simulink model "OFDMTxRx2211"  (R2017b)
settings: Solver=VariableStepAuto  StartTime=0.0  StopTime=10.0  RelTol=1e-3
InitFcn:
  | Ts = 1e-6;
  | simParams.Ts = Ts;
  | simParams.TsTx = Ts;
  | simParams.TsRx = Ts;
  | simParams.nFFT = 1024;
  | simParams.lengthCP = 128;
  | nFFT = simParams.nFFT;
  | simParams.NSubcarriers = 398;
  | simParams.windowing = 16;
undefined symbols (not defined in the file): fft_size, i
libraries: hdlsllib x49, simulink x39, simulink_need_slupdate x12, dspmathops x4, dspxfrm3 x3, dspsigops x2, commdigbbndam3 x1, commseqgen3 x1
(part 1 of 3)
settings Model: PauseTimes=1  NumberOfSteps=100  Creator=Pigrit  LastModifiedBy=trainee

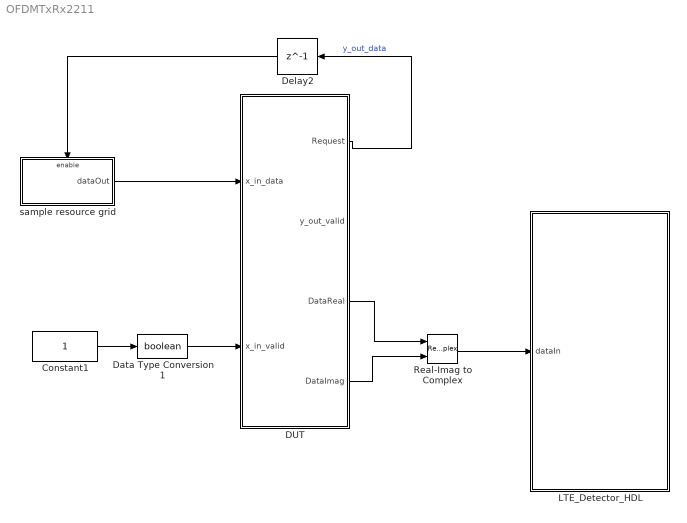
== system OFDMTxRx2211 ==
  Constant1 : Constant  OutDataTypeStr=boolean  SampleTime=simParams.Ts
  DUT : Subsystem  TreatAsAtomicUnit=on
  Data Type Conversion1 : DataTypeConversion  OutDataTypeStr=boolean
  Delay2 : Delay  DelayLength=1  InitialCondition=0  InputProcessing=Columns as channels (frame based)
  LTE_Detector_HDL : Subsystem
  Real-Imag to Complex : RealImagToComplex
  sample resource grid : Subsystem
  wires:
  DUT/3(DataReal) -> Real-Imag to Complex/1
  Delay2/1 -> sample resource grid/Enable
  Data Type Conversion1/1 -> DUT/2(x_in_valid)
  Constant1/1 -> Data Type Conversion1/1
  DUT/1(Request) -> Delay2/1  "y_out_data"
  sample resource grid/1(dataOut) -> DUT/1(x_in_data)
  DUT/4(DataImag) -> Real-Imag to Complex/2
  Real-Imag to Complex/1 -> LTE_Detector_HDL/1(dataIn)

== system OFDMTxRx2211/DUT ==
  x_in_data : Inport
  x_in_valid : Inport  Port=2
  "symmetric " : Subsystem
  Request : Outport
  y_out_valid : Outport  Port=2
  DataReal : Outport  Port=3
  DataImag : Outport  Port=4
  wires:
  x_in_valid/1 -> "symmetric "/Enable, y_out_valid/1
  x_in_data/1 -> "symmetric "/1(x_in)
  "symmetric "/1(y_out) -> Request/1
  "symmetric "/2(Data1) -> DataReal/1
  "symmetric "/3(Data2) -> DataImag/1

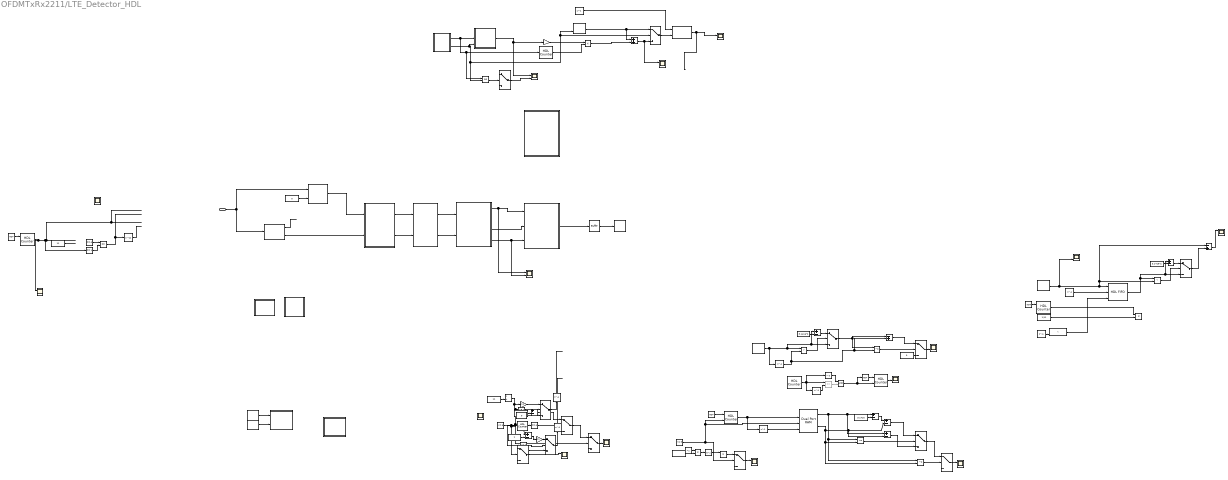
== system OFDMTxRx2211/LTE_Detector_HDL ==
  dataIn : Inport
  Add{,1..4,6,8} (7 alike) : Sum  Inputs=+-
  Add5 : Sum  Inputs=-+
  Add7 : Sum  Inputs=-+
  Add9 : Sum
  AmpAndAngle : Subsystem
  Buffer : Buffer  N=1000  OutputFrames=off
  Compare To Constant : simulink/Logic and Bit Operations/Compare To Constant  relop=>=  const=5  OutDataTypeStr=boolean
  Compare To Constant1 : simulink/Logic and Bit Operations/Compare To Constant  relop===  const=0  OutDataTypeStr=boolean
  Compare To Constant2 : simulink/Logic and Bit Operations/Compare To Constant  relop===  const=1  OutDataTypeStr=boolean
  Compare To Constant3 : simulink/Logic and Bit Operations/Compare To Constant  relop=>=  const=5  OutDataTypeStr=boolean
  Compare To Constant4 : simulink/Logic and Bit Operations/Compare To Constant  relop=>  const=0  OutDataTypeStr=boolean
  Compare To Constant5 : simulink/Logic and Bit Operations/Compare To Constant  relop===  const=0  OutDataTypeStr=boolean
  Compare To Constant6 : simulink/Logic and Bit Operations/Compare To Constant  relop=>=  const=1  OutDataTypeStr=boolean
  Compare To Constant7 : simulink/Logic and Bit Operations/Compare To Constant  relop=>=  const=1  OutDataTypeStr=boolean
  Constant1 : Constant  Value=3.1416  OutDataTypeStr=double  SampleTime=simParams.Ts
  Constant10 : Constant  Value=0  OutDataTypeStr=uint8  SampleTime=simParams.Ts
  Constant11 : Constant  OutDataTypeStr=double  SampleTime=simParams.Ts
  Constant12 : Constant  Value=11  OutDataTypeStr=uint8  SampleTime=simParams.Ts
  Constant2 : Constant  Value=complex(0+i)  SampleTime=simParams.Ts
  Constant3 : Constant  Value=3.1416  OutDataTypeStr=double  SampleTime=simParams.Ts
  Constant4 : Constant  Value=3.1416*2  OutDataTypeStr=double  SampleTime=simParams.Ts
  Constant5 : Constant  Value=0  OutDataTypeStr=double  SampleTime=simParams.Ts
  Constant6 : Constant  Value=1/11  SampleTime=simParams.Ts
  Constant7 : Constant  Value=3.1416*2  OutDataTypeStr=double  SampleTime=simParams.Ts
  Constant8 : Constant  Value=11  OutDataTypeStr=int16  SampleTime=simParams.Ts
  Constant9 : Constant  Value=0  OutDataTypeStr=int8  SampleTime=simParams.Ts
  Constellation Diagram : ConstellationDiagram
  Delay1 : Delay  DelayLength=1  InitialCondition=0  InputProcessing=Columns as channels (frame based)
  Delay{2..3,6..9} (6 alike) : Delay  DelayLength=1  InitialCondition=0  UseCircularBuffer=on
  Delay4 : Delay  DelayLength=1  InitialCondition=0  InputProcessing=Columns as channels (frame based)
  Delay5 : Delay  DelayLength=11  InitialCondition=0  InputProcessing=Columns as channels (frame based)
  Divide : Product  Inputs=*/  OutDataTypeStr=uint8  SaturateOnIntegerOverflow=on  RndMeth=Zero
  Dual Port RAM : hdlsllib/HDL RAMs/Dual Port RAM  ram_size=8
      settings: SourceProductName=HDL Coder  SourceProductBaseCode=HD
  FFT : Subsystem
  Frequency_Correction : Subsystem
  Frequency_Correction1 : Subsystem
  Frequency_Estimation : Subsystem
  Frequency_Estimation1 : Subsystem
  Gain : Gain  Gain=11  OutDataTypeStr=uint8
  Gain1 : Gain  Gain=11  OutDataTypeStr=uint8
  Gain2 : Gain  Gain=1/10
  HDL Counter : hdlsllib/Sources/HDL Counter  CountType=Count limited  CountInit=0  CountStep=1  CountMax=1  CountFromType=Initial value  CountFrom=0  CountResetPort=off  CountLoadPort=off  CountEnbPort=on  CountDirPort=off  CountDataType=Unsigned  CountWordLen=1  CountFracLen=0  CountSampTime=1
      settings: SourceProductBaseCode=HD
  HDL Counter1 : hdlsllib/Sources/HDL Counter  CountType=Count limited  CountInit=1  CountStep=1  CountMax=60  CountFromType=Initial value  CountFrom=1  CountResetPort=on  CountLoadPort=off  CountEnbPort=on  CountDirPort=off  CountDataType=Unsigned  CountWordLen=8  CountFracLen=0  CountSampTime=1
      settings: SourceProductBaseCode=HD
  HDL Counter2 : hdlsllib/Sources/HDL Counter  CountType=Count limited  CountInit=0  CountStep=1  CountMax=60  CountFromType=Initial value  CountFrom=0  CountResetPort=on  CountLoadPort=off  CountEnbPort=on  CountDirPort=off  CountDataType=Unsigned  CountWordLen=8  CountFracLen=0  CountSampTime=1
      settings: SourceProductBaseCode=HD
  HDL Counter3 : hdlsllib/Sources/HDL Counter  CountType=Count limited  CountInit=0  CountStep=1  CountMax=1024  CountFromType=Initial value  CountFrom=0  CountResetPort=on  CountLoadPort=off  CountEnbPort=on  CountDirPort=off  CountDataType=Unsigned  CountWordLen=16  CountFracLen=0  CountSampTime=1
      settings: SourceProductBaseCode=HD
  HDL Counter4 : hdlsllib/Sources/HDL Counter  CountType=Count limited  CountInit=0  CountStep=1  CountMax=40  CountFromType=Initial value  CountFrom=0  CountResetPort=off  CountLoadPort=off  CountEnbPort=on  CountDirPort=off  CountDataType=Unsigned  CountWordLen=8  CountFracLen=0  CountSampTime=1
      settings: SourceProductBaseCode=HD
  HDL Counter5 : hdlsllib/Sources/HDL Counter  CountType=Count limited  CountInit=0  CountStep=1  CountMax=40  CountFromType=Initial value  CountFrom=0  CountResetPort=on  CountLoadPort=off  CountEnbPort=on  CountDirPort=off  CountDataType=Unsigned  CountWordLen=8  CountFracLen=0  CountSampTime=1
      settings: SourceProductBaseCode=HD
  HDL Counter7 : hdlsllib/Sources/HDL Counter  CountType=Count limited  CountInit=0  CountStep=1  CountMax=9  CountFromType=Initial value  CountFrom=0  CountResetPort=off  CountLoadPort=off  CountEnbPort=on  CountDirPort=off  CountDataType=Unsigned  CountWordLen=8  CountFracLen=0  CountSampTime=1
      settings: SourceProductBaseCode=HD
  HDL FIFO : hdlsllib/HDL RAMs/HDL FIFO  fifo_size=40  ratio=1  push_msg=Warning  pop_msg=Warning  show_empty=off  show_full=off  show_num=off
      settings: SourceProductName=HDL Coder  SourceProductBaseCode=HD
  Logical Operator1 : Logic  Operator=NOT  IconShape=distinctive  AllPortsSameDT=off  OutDataTypeStr=boolean
  Logical Operator2 : Logic  Operator=NOT  IconShape=distinctive  AllPortsSameDT=off  OutDataTypeStr=boolean
  Logical Operator3 : Logic  Operator=OR  AllPortsSameDT=off  OutDataTypeStr=boolean
  Logical Operator4 : Logic  Operator=OR  AllPortsSameDT=off  OutDataTypeStr=boolean
  Logical Operator6 : Logic  AllPortsSameDT=off  OutDataTypeStr=boolean
  Logical Operator7 : Logic  Operator=NOT  Inputs=1  AllPortsSameDT=off  OutDataTypeStr=boolean
  Logical Operator8 : Logic  Operator=NOT  AllPortsSameDT=off  OutDataTypeStr=boolean
  Number of subcarriers : Constant  Value=0  OutDataTypeStr=fixdt(0,12,0)  SampleTime=Ts
  Pow : Math  RndMeth=Zero  SaturateOnIntegerOverflow=on
  Product{,1..3} (4 alike) : Product
  Relational Operator : RelationalOperator  Operator=~=  OutDataTypeStr=boolean  RndMeth=Nearest
  Relational Operator1 : RelationalOperator  Operator=<=  OutDataTypeStr=boolean  RndMeth=Nearest
  Relational Operator2 : RelationalOperator  Operator=>  OutDataTypeStr=boolean  RndMeth=Nearest
  Relational Operator3 : RelationalOperator  Operator=~=  OutDataTypeStr=boolean  RndMeth=Nearest
  Relational Operator4 : RelationalOperator  Operator=<  OutDataTypeStr=boolean  RndMeth=Nearest
  Relational Operator5 : RelationalOperator  Commented=on  Operator===  OutDataTypeStr=boolean  RndMeth=Nearest
  Relational Operator6 : RelationalOperator  Operator=<  OutDataTypeStr=boolean  RndMeth=Nearest
  Scope{1..3,5..8,11..15} (12 alike) : Scope  NumInputPorts=2
  Scope10 : Scope  NumInputPorts=3
  Scope4 : Scope
  Scope9 : Scope  NumInputPorts=3
  Subsystem1 : Subsystem
  Subsystem2 : Subsystem
  Switch{1..13} (13 alike) : Switch  Criteria=u2 ~= 0
  Unary Minus : UnaryMinus
  Unit Delay Enabled Synchronous{1..4,6} (5 alike) : hdlsllib/Discrete/Unit Delay Enabled Synchronous  InitialCondition=0.0  SampleTime=-1
      settings: SourceProductName=HDL Coder  SourceProductBaseCode=HD
  Подкрутка фазы1 : Subsystem
  Подстройка фаз по пилотным : Subsystem
  "Рабочая версия с недокрученной фазой " : Subsystem
  Стробирование сигнала на nFFT отсчетов : Subsystem
  Устранение 2pi неопределенности и вычисление разности фаз : Subsystem
  Устранение 2pi неопределенности и вычисление разности фаз2 : Subsystem
  wires:
  Frequency_Estimation1/1(freqEst) -> ?
  Frequency_Correction1/1(dataOut) -> Стробирование сигнала на nFFT отсчетов/1(In1)
  Frequency_Estimation1/2(MiddlePoint) -> Стробирование сигнала на nFFT отсчетов/2(In2)
  Стробирование сигнала на nFFT отсчетов/1(dataOut) -> FFT/1(dataIn)
  Стробирование сигнала на nFFT отсчетов/2(ValidOut) -> FFT/2(validIn)
  Switch1/1 -> Switch2/1
  Switch2/1 -> Scope4/1
  ? -> Switch1/3, Add/1, Switch3/1
  Compare To Constant/1 -> Switch2/2, Switch3/2, HDL Counter/1
  Switch3/1 -> Scope2/1
  Compare To Constant1/1 -> Switch1/2
  Add/1 -> Switch1/1
  Constant1/1 -> Add/2
  HDL Counter/1 -> Compare To Constant1/1
  ? -> Scope2/2, Compare To Constant/1
  Switch7/1 -> Scope1/1
  Pow/1 -> Product1/1
  ? -> Dual Port RAM/1, Unary Minus/1
  ? -> Compare To Constant3/1
  Unary Minus/1 -> Product/1
  Logical Operator2/1 -> HDL Counter2/1
  Add1/1 -> Add2/1
  Relational Operator1/1 -> Switch6/2
  Constant3/1 -> Add1/2
  Add3/1 -> Switch6/3
  Relational Operator/1 -> Switch7/2
  Compare To Constant3/1 -> Dual Port RAM/3, HDL Counter2/2, Switch5/2
  Add2/1 -> Switch6/1
  Delay2/1 -> Dual Port RAM/4
  Constant2/1 -> Product/2
  Switch5/1 -> Scope3/1
  ? -> Product1/2
  Dual Port RAM/2 -> Relational Operator1/2, Relational Operator/2, Add3/2, Add2/2
  Dual Port RAM/1 -> Add3/1, Add1/1, Relational Operator1/1, Relational Operator/1
  Product1/1 -> Switch5/1
  Switch6/1 -> Switch7/1
  HDL Counter2/1 -> Dual Port RAM/2, Delay2/1
  ? -> Logical Operator2/1, Scope3/2
  Product/1 -> Pow/1
  FFT/1(dataOut) -> AmpAndAngle/1(In1)
  FFT/2(validOut) -> AmpAndAngle/2(In2)
  Logical Operator6/1 -> Logical Operator7/1, HDL Counter5/2
  Relational Operator5/1 -> Logical Operator6/2
  Compare To Constant4/1 -> Logical Operator6/1
  Delay6/1 -> Relational Operator5/2
  HDL Counter4/1 -> Compare To Constant4/1, Relational Operator5/1, Delay6/1
  Switch9/1 -> Scope5/2
  Switch8/1 -> Add5/1, Relational Operator3/1
  Constant5/1 -> Switch9/3
  Unit Delay Enabled Synchronous1/1 -> Add4/1, Switch8/3, Relational Operator2/1, Delay3/1
  Relational Operator3/1 -> Switch9/2
  Relational Operator2/1 -> Switch8/2
  Constant4/1 -> Add4/2
  Logical Operator7/1 -> HDL Counter5/1
  Add4/1 -> Switch8/1
  Add5/1 -> Switch9/1
  HDL Counter5/1 -> Scope7/2
  ? -> HDL Counter4/1, Unit Delay Enabled Synchronous1/2
  Delay3/1 -> Add5/2, Relational Operator3/2, Relational Operator2/2
  ? -> Delay1/1
  HDL FIFO/1 -> Add6/1, Switch4/3, Relational Operator6/1
  ? -> Unit Delay Enabled Synchronous2/2
  Logical Operator1/1 -> HDL Counter1/1
  ? -> Unit Delay Enabled Synchronous2/1
  Constant7/1 -> Add6/2
  Relational Operator6/1 -> Switch4/2
  Add7/1 -> Scope6/1
  ? -> Scope6/2
  ? -> HDL Counter1/2
  Add6/1 -> Switch4/1
  Delay1/1 -> Relational Operator4/2
  Constant6/1 -> Product2/2
  Unit Delay Enabled Synchronous2/1 -> Scope8/2, Add7/1, Relational Operator6/2, HDL FIFO/1
  ? -> Relational Operator4/1
  ? -> Delay4/1
  Switch4/1 -> Add7/2
  Delay4/1 -> HDL FIFO/2
  HDL Counter1/1 -> Product2/1
  Relational Operator4/1 -> HDL FIFO/3
  Unit Delay Enabled Synchronous3/1 -> Устранение 2pi неопределенности и вычисление разности фаз/2("Фаза \"правого\" пилота")
  Unit Delay Enabled Synchronous4/1 -> Устранение 2pi неопределенности и вычисление разности фаз/1("Фаза \"левого\" пилота")
  ? -> Unit Delay Enabled Synchronous3/1
  ? -> Unit Delay Enabled Synchronous4/1
  Constant8/1 -> ?
  ? -> Compare To Constant5/1
  Compare To Constant2/1 -> Logical Operator3/2
  ? -> Logical Operator8/1, Scope10/2, HDL Counter3/2
  ? -> ?
  Delay5/1 -> ?
  ? -> Scope9/1
  Logical Operator8/1 -> HDL Counter3/1
  Logical Operator3/1 -> Delay5/1
  HDL Counter3/1 -> Scope10/1, Compare To Constant2/1
  Compare To Constant5/1 -> Logical Operator3/1
  Delay7/1 -> ?
  Add8/1 -> Gain1/1
  Compare To Constant6/1 -> Switch10/2
  Gain/1 -> Switch10/1
  Constant9/1 -> Switch10/3
  Switch11/1 -> Delay7/1
  Delay8/1 -> ?
  Constant10/1 -> Switch11/3
  Constant12/1 -> Divide/2
  ? -> Divide/1
  Divide/1 -> Gain/1, Add8/1, Compare To Constant7/1, Compare To Constant6/1
  Constant11/1 -> Add8/2
  Compare To Constant7/1 -> Switch11/2
  Switch10/1 -> Delay8/1
  Gain1/1 -> Switch11/1
  ? -> Delay9/1
  Подкрутка фазы1/1(Out1) -> Scope12/1
  Add9/1 -> Scope15/1, Switch12/3
  Gain2/1 -> Product3/1
  Unit Delay Enabled Synchronous6/1 -> Add9/1, Switch12/1
  Subsystem2/1("Passe diff ") -> Scope13/1, Gain2/1
  Subsystem1/2(IndexPilot) -> Logical Operator4/2, Unit Delay Enabled Synchronous6/2, Switch12/2, Subsystem2/3("Index Pil ")
  Subsystem1/1(InformIndex) -> Logical Operator4/1, HDL Counter7/1, Subsystem2/2(Index Inf)
  Delay9/1 -> Подкрутка фазы1/1(PuuuSii)
  HDL Counter7/1 -> Product3/2
  ? -> Switch13/1, Unit Delay Enabled Synchronous6/1, Subsystem2/1(Pilot Phase)
  Switch13/1 -> Scope13/2
  Product3/1 -> Add9/2
  Logical Operator4/1 -> Switch13/2
  Switch12/1 -> Подкрутка фазы1/2("DifPhase ")
  Buffer/1 -> Constellation Diagram/1
  AmpAndAngle/3(AngOut) -> Подстройка фаз по пилотным/2(AngIn)
  AmpAndAngle/4(ValidOut) -> Scope14/2, Подстройка фаз по пилотным/3("ValidIn ")
  Подстройка фаз по пилотным/1(Out1) -> Buffer/1
  AmpAndAngle/1("PureSig ") -> Scope14/1, Подстройка фаз по пилотным/1(PureSigIn)
  dataIn/1 -> Frequency_Correction1/1(dataIn), Frequency_Estimation1/1(data)
  Number of subcarriers/1 -> Frequency_Correction1/2(freq)

== system OFDMTxRx2211/sample resource grid ==
  request1 : EnablePort
  PN Sequence Generator : commseqgen3/PN Sequence Generator  poly='z^23+z^21+z^17 + z^11 + z^5 +1'  ini_sta=[0 1 1 0 0 1 0 0 0 0 1 0 1 1 0 0 1 0 0 1 0 0 1]  outBitMaskSource=Dialog parameter  shift=0  outVarSiz=off  maxOutSizeMode=Dialog parameter  maxOutSize=[10 1]  Ts=simParams.Ts  sampPerFrame=1  reset=off  bitPackedOutputs=on  outDataType=boolean  numPackedBits=2  bitPackDataSigned=off  bitPackedOutDType=Smallest integer
      settings: SourceProductName=Communications System Toolbox
  dataOut : Outport
  wires:
  PN Sequence Generator/1 -> dataOut/1

== system OFDMTxRx2211/DUT/symmetric  ==
  x_in : Inport
  Enable : EnablePort
  Add CP and windowing : Subsystem
  Complex to Real-Imag : ComplexToRealImag
  IFFT : Subsystem
  Scope : Scope  NumInputPorts=2
  Scope1 : Scope  NumInputPorts=2
  fORM1 : Subsystem
  y_out1 : Scope  NumInputPorts=2
  "Сдвиг в симметричный вид " : Subsystem
  y_out : Outport  InitialOutput=0
  Data1 : Outport  Port=2  InitialOutput=0
  Data2 : Outport  Port=3  InitialOutput=0
  wires:
  fORM1/1(dataRequest) -> y_out/1
  x_in/1 -> fORM1/1(dataIn)
  Add CP and windowing/1(Out1) -> Complex to Real-Imag/1
  Complex to Real-Imag/1 -> Data2/1
  IFFT/1(dataOut) -> Scope/1, Add CP and windowing/1(In1)
  Complex to Real-Imag/2 -> Data1/1
  "Сдвиг в симметричный вид "/1(dataOut) -> Scope1/1, IFFT/1(dataIn)
  "Сдвиг в симметричный вид "/2(validOut) -> Scope1/2, IFFT/2(validIn)
  IFFT/2(validOut) -> Scope/2, Add CP and windowing/2(In2)
  fORM1/2(dataOut) -> y_out1/1, "Сдвиг в симметричный вид "/1(dataIn)
  fORM1/3(validOut) -> y_out1/2, "Сдвиг в симметричный вид "/2(validIn)

== system OFDMTxRx2211/LTE_Detector_HDL/AmpAndAngle ==
  In1 : Inport
  In2 : Inport  Port=2
  Compare To Constant2 : simulink/Logic and Bit Operations/Compare To Constant  relop=<  const=512  OutDataTypeStr=boolean
  Delay1 : Delay  DelayLength=512  InitialCondition=0  InputProcessing=Columns as channels (frame based)
  Delay2 : Delay  DelayLength=22  InitialCondition=0  InputProcessing=Columns as channels (frame based)
  Delay4 : Delay  DelayLength=1024  InitialCondition=0  InputProcessing=Columns as channels (frame based)
  HDL Counter1 : hdlsllib/Sources/HDL Counter  CountType=Count limited  CountInit=0  CountStep=1  CountMax=1023  CountFromType=Initial value  CountFrom=0  CountResetPort=on  CountLoadPort=off  CountEnbPort=on  CountDirPort=off  CountDataType=Unsigned  CountWordLen=11  CountFracLen=0  CountSampTime=1
      settings: SourceProductBaseCode=HD
  Logical Operator1 : Logic  Operator=NOT  IconShape=distinctive  AllPortsSameDT=off  OutDataTypeStr=boolean
  Rect_to_Polar : Subsystem
  Signal Specification1 : SignalSpecification  Dimensions=1
  Switch4 : Switch  Criteria=u2 ~= 0
  "PureSig " : Outport
  MagOut : Outport  Port=2
  AngOut : Outport  Port=3
  ValidOut : Outport  Port=4
  wires:
  Delay4/1 -> Switch4/3
  Compare To Constant2/1 -> Switch4/2
  HDL Counter1/1 -> Compare To Constant2/1
  Logical Operator1/1 -> HDL Counter1/1
  Switch4/1 -> Delay2/1, Signal Specification1/1
  Delay1/1 -> Logical Operator1/1, HDL Counter1/2, Rect_to_Polar/2("ValidIn ")
  In2/1 -> Delay1/1
  In1/1 -> Switch4/1, Delay4/1
  Rect_to_Polar/3(validOut) -> ValidOut/1
  Rect_to_Polar/1(magOut) -> MagOut/1
  Delay2/1 -> "PureSig "/1
  Rect_to_Polar/2(angleOut) -> AngOut/1
  Signal Specification1/1 -> Rect_to_Polar/1(dataIn)

== system OFDMTxRx2211/LTE_Detector_HDL/FFT ==
  note: Set input of FFT to input wordlength + FFT growth to allow
      | the output of the FFT to scale. Maximum bit growth is equal
      | to log2(nFFT).
  dataIn : Inport
  validIn : Inport  Port=2
  Data Type Conversion : DataTypeConversion  OutDataTypeStr=fixdt(1,18,10)  RndMeth=Round
  Delay{1..2,4..5} (4 alike) : Delay  DelayLength=1  InitialCondition=0  InputProcessing=Columns as channels (frame based)
  FFT HDL Optimized : dspxfrm3/FFT HDL Optimized  FFTLength=1024  Architecture=Streaming Radix 2^2  ComplexMultiplication=Use 3 multipliers and 5 adders  BitReversedOutput=off  BitReversedInput=off  Normalize=off  SimulateUsing=Code generation  RoundingMethod=Floor  ResetInputPort=off  StartOutputPort=off  EndOutputPort=off
      settings: SourceProductName=DSP System Toolbox  SourceProductBaseCode=DS
  Signal Specification : SignalSpecification  Dimensions=1
  Signal Specification1 : SignalSpecification  Dimensions=1
  dataOut : Outport
  validOut : Outport  Port=2
  wires:
  Signal Specification1/1 -> FFT HDL Optimized/2
  Signal Specification/1 -> FFT HDL Optimized/1
  FFT HDL Optimized/2 -> Delay5/1
  FFT HDL Optimized/1 -> Delay4/1
  Delay4/1 -> Data Type Conversion/1
  Delay2/1 -> Signal Specification1/1
  dataIn/1 -> Delay1/1
  validIn/1 -> Delay2/1
  Delay1/1 -> Signal Specification/1
  Data Type Conversion/1 -> dataOut/1
  Delay5/1 -> validOut/1

== system OFDMTxRx2211/LTE_Detector_HDL/Frequency_Correction ==
  note: This subsystem corrects the frequency offset using an Numerically Controller Oscillator (NCO) and a conjugate multiplication.
  dataIn : Inport
  freq : Inport  Port=2
  Data Type Conversion : DataTypeConversion  OutDataTypeStr=fixdt(1,16,15)  RndMeth=Nearest
  Delay{1..6} (6 alike) : Delay  DelayLength=1  InitialCondition=0  UseCircularBuffer=on
  Gain : Gain  Gain=2^9  OutDataTypeStr=int16
  NCO HDL Optimized : dspsigops/NCO HDL Optimized  PhaseIncrementSource=Input port  PhaseIncrement=100  PhaseOffsetSource=Property  PhaseOffset=0  DitherSource=Property  NumDitherBits=4  PhaseQuantization=on  NumQuantizerAccumulatorBits=12  LUTCompress=on  ResetAction=off  ValidInputPort=off  Waveform=Complex exponential  PhasePort=off  SimulateUsing=Code generation  AccumulatorWL=16  OutputDataType=Binary point scaling  OutputWL=16  OutputFL=14
      settings: SourceProductName=DSP System Toolbox  SourceProductBaseCode=DS
  Product1 : Product
  Scope : Scope  NumInputPorts=2
  Signal Spec : SignalSpecification  Dimensions=1
  Unit Delay Enabled : simulink_need_slupdate/Unit Delay Enabled  vinit=0.0  tsamp=-1
      settings: SourceProductName=Simulink  SourceProductBaseCode=SL
  complexConjugate : Math  Operator=conj  SaturateOnIntegerOverflow=on
  dataOut : Outport
  wires:
  complexConjugate/1 -> Delay3/1
  NCO HDL Optimized/2 -> Unit Delay Enabled/2
  dataIn/1 -> Delay2/1
  Product1/1 -> Delay4/1
  NCO HDL Optimized/1 -> Unit Delay Enabled/1
  Unit Delay Enabled/1 -> complexConjugate/1
  Data Type Conversion/1 -> Delay1/1
  Delay2/1 -> Scope/2, Product1/1
  Delay1/1 -> dataOut/1
  Delay4/1 -> Data Type Conversion/1
  Delay3/1 -> Scope/1, Product1/2
  Gain/1 -> Delay5/1
  freq/1 -> Delay6/1
  Delay6/1 -> Gain/1
  Signal Spec/1 -> NCO HDL Optimized/1
  Delay5/1 -> Signal Spec/1

== system OFDMTxRx2211/LTE_Detector_HDL/Frequency_Correction1 ==
  note: This subsystem corrects the frequency offset using an Numerically Controller Oscillator (NCO) and a conjugate multiplication.
  dataIn : Inport
  freq : Inport  Port=2
  Data Type Conversion : DataTypeConversion  OutDataTypeStr=fixdt(1,16,15)  RndMeth=Nearest
  Delay{1..6} (6 alike) : Delay  DelayLength=1  InitialCondition=0  UseCircularBuffer=on
  Gain : Gain  Gain=2^9  OutDataTypeStr=int16
  NCO HDL Optimized : dspsigops/NCO HDL Optimized  PhaseIncrementSource=Input port  PhaseIncrement=100  PhaseOffsetSource=Property  PhaseOffset=0  DitherSource=Property  NumDitherBits=4  PhaseQuantization=on  NumQuantizerAccumulatorBits=12  LUTCompress=on  ResetAction=off  ValidInputPort=off  Waveform=Complex exponential  PhasePort=off  SimulateUsing=Code generation  AccumulatorWL=16  OutputDataType=Binary point scaling  OutputWL=16  OutputFL=14
      settings: SourceProductName=DSP System Toolbox  SourceProductBaseCode=DS
  Product1 : Product
  Scope : Scope  NumInputPorts=2
  Signal Spec : SignalSpecification  Dimensions=1
  Unit Delay Enabled : simulink_need_slupdate/Unit Delay Enabled  vinit=0.0  tsamp=-1
      settings: SourceProductName=Simulink  SourceProductBaseCode=SL
  complexConjugate : Math  Operator=conj  SaturateOnIntegerOverflow=on
  dataOut : Outport
  wires:
  complexConjugate/1 -> Delay3/1
  NCO HDL Optimized/2 -> Unit Delay Enabled/2
  dataIn/1 -> Delay2/1
  Product1/1 -> Delay4/1
  NCO HDL Optimized/1 -> Unit Delay Enabled/1
  Unit Delay Enabled/1 -> complexConjugate/1
  Data Type Conversion/1 -> Delay1/1
  Delay2/1 -> Scope/2, Product1/1
  Delay1/1 -> dataOut/1
  Delay4/1 -> Data Type Conversion/1
  Delay3/1 -> Scope/1, Product1/2
  Gain/1 -> Delay5/1
  freq/1 -> Delay6/1
  Delay6/1 -> Gain/1
  Signal Spec/1 -> NCO HDL Optimized/1
  Delay5/1 -> Signal Spec/1

== system OFDMTxRx2211/LTE_Detector_HDL/Frequency_Estimation ==
  data : Inport
  Angle_Filter : Subsystem
  Angle_at_Maximum : Subsystem
  Cyclic_Prefix_Correlator : Subsystem
  Delay14 : Delay  DelayLength=30  InitialCondition=0  UseCircularBuffer=on
  Rect_to_Polar : Subsystem
  Scope1 : Scope  NumInputPorts=2
  freqEst : Outport
  MiddlePoint : Outport  Port=2
  wires:
  Angle_at_Maximum/1(angleOut) -> Angle_Filter/1(angleIn)
  Cyclic_Prefix_Correlator/1(corrOut) -> Scope1/2, Rect_to_Polar/1(dataIn)
  Angle_at_Maximum/2(validOut) -> Delay14/1, MiddlePoint/1, Angle_Filter/2(en)
  Angle_Filter/1(angleOut) -> freqEst/1
  data/1 -> Cyclic_Prefix_Correlator/1(dataIn)
  Delay14/1 -> Scope1/1
  Rect_to_Polar/1(magOut) -> Angle_at_Maximum/1(MagIn)
  Rect_to_Polar/2(angleOut) -> Angle_at_Maximum/2(AngleIn)
  Rect_to_Polar/3(validOut) -> Angle_at_Maximum/3(ValidIn)

== system OFDMTxRx2211/LTE_Detector_HDL/Frequency_Estimation1 ==
  data : Inport
  Angle_Filter : Subsystem
  Angle_at_Maximum : Subsystem
  Cyclic_Prefix_Correlator : Subsystem
  Delay14 : Delay  DelayLength=30  InitialCondition=0  UseCircularBuffer=on
  Rect_to_Polar : Subsystem
  Scope1 : Scope  NumInputPorts=2
  freqEst : Outport
  MiddlePoint : Outport  Port=2
  wires:
  Rect_to_Polar/3(validOut) -> Angle_at_Maximum/3(validIn)
  Angle_at_Maximum/1(angleOut) -> Angle_Filter/1(angleIn)
  Rect_to_Polar/1(magOut) -> Angle_at_Maximum/1(magIn)
  Cyclic_Prefix_Correlator/1(corrOut) -> Scope1/2, Rect_to_Polar/1(dataIn)
  Angle_at_Maximum/2(ValidOut) -> Delay14/1, MiddlePoint/1, Angle_Filter/2(en)
  Rect_to_Polar/2(angleOut) -> Angle_at_Maximum/2(angleIn)
  Angle_Filter/1(angleOut) -> freqEst/1
  data/1 -> Cyclic_Prefix_Correlator/1(dataIn)
  Delay14/1 -> Scope1/1

== system OFDMTxRx2211/LTE_Detector_HDL/Subsystem1 ==
  In1 : Inport
  AND : Logic  IconShape=distinctive  AllPortsSameDT=off  OutDataTypeStr=boolean
  Abs : Abs
  Add6 : Sum  Inputs=+-  OutDataTypeStr=fixdt(1,16,0)
  Compare To Constant5 : simulink/Logic and Bit Operations/Compare To Constant  relop===  const=1  OutDataTypeStr=boolean
  Compare To Zero : simulink/Logic and Bit Operations/Compare To Zero  relop=~=  OutDataTypeStr=boolean
  Constant6 : Constant  Value=11  OutDataTypeStr=int16  SampleTime=simParams.Ts
  FFT Size : Constant  Value=nFFT  OutDataTypeStr=fixdt(0,ceil(log2(simParams.nFFT))+1,0)  SampleTime=Ts
  FFT Size / 2 : ArithShift  BitShiftNumber=1  BitShiftDirection=Right
  HDL Counter3 : hdlsllib/Sources/HDL Counter  CountType=Count limited  CountInit=0  CountStep=1  CountMax=1023  CountFromType=Initial value  CountFrom=0  CountResetPort=off  CountLoadPort=off  CountEnbPort=on  CountDirPort=off  CountDataType=Unsigned  CountWordLen=11  CountFracLen=0  CountSampTime=1
      settings: SourceProductBaseCode=HD
  Logical Operator : Logic  AllPortsSameDT=off  OutDataTypeStr=boolean
  Logical Operator3 : Logic  Operator=NOT  Inputs=1  AllPortsSameDT=off  OutDataTypeStr=boolean
  Logical Operator4 : Logic  AllPortsSameDT=off  OutDataTypeStr=boolean
  Math Function : Math  Operator=mod  RndMeth=Zero  SaturateOnIntegerOverflow=on
  NSubcarriers / 2 : ArithShift  BitShiftNumber=1  BitShiftDirection=Right
  Number of subcarriers : Constant  Value=simParams.NSubcarriers  OutDataTypeStr=fixdt(0,12,0)  SampleTime=Ts
  Relational Operator4 : RelationalOperator  Operator=<=  OutDataTypeStr=boolean  RndMeth=Nearest
  InformIndex : Outport
  IndexPilot : Outport  Port=2
  wires:
  In1/1 -> HDL Counter3/1
  HDL Counter3/1 -> Add6/2
  FFT Size/1 -> FFT Size / 2/1
  Logical Operator/1 -> InformIndex/1
  Constant6/1 -> Math Function/2
  AND/1 -> Logical Operator4/2, Logical Operator/2
  Number of subcarriers/1 -> NSubcarriers / 2/1
  Add6/1 -> Abs/1
  Logical Operator3/1 -> Logical Operator/1
  Abs/1 -> Relational Operator4/1, Compare To Zero/1, Math Function/1
  NSubcarriers / 2/1 -> Relational Operator4/2
  FFT Size / 2/1 -> Add6/1
  Compare To Zero/1 -> AND/1
  Math Function/1 -> Compare To Constant5/1
  Relational Operator4/1 -> AND/2
  Logical Operator4/1 -> IndexPilot/1
  Compare To Constant5/1 -> Logical Operator4/1, Logical Operator3/1

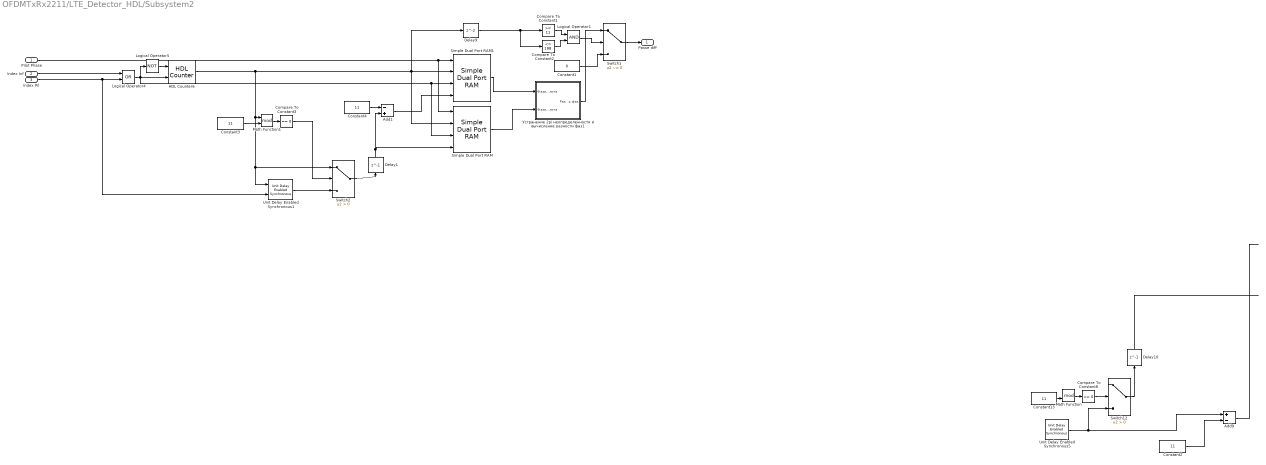
== system OFDMTxRx2211/LTE_Detector_HDL/Subsystem2 ==
  Pilot Phase : Inport
  Index Inf : Inport  Port=2
  "Index Pil " : Inport  Port=3
  Add1 : Sum  Inputs=-+
  Add9 : Sum  Inputs=+-
  Compare To Constant1 : simulink/Logic and Bit Operations/Compare To Constant  relop=>=  const=11  OutDataTypeStr=boolean
  Compare To Constant2 : simulink/Logic and Bit Operations/Compare To Constant  relop=<=  const=198  OutDataTypeStr=boolean
  Compare To Constant3 : simulink/Logic and Bit Operations/Compare To Constant  relop===  const=0  OutDataTypeStr=boolean
  Compare To Constant8 : simulink/Logic and Bit Operations/Compare To Constant  relop===  const=0  OutDataTypeStr=boolean
  Constant1 : Constant  Value=0  OutDataTypeStr=uint8  SampleTime=simParams.Ts
  Constant{2..4,13} (4 alike) : Constant  Value=11  OutDataTypeStr=uint8  SampleTime=simParams.Ts
  Delay1 : Delay  DelayLength=1  InitialCondition=0  UseCircularBuffer=on
  Delay10 : Delay  DelayLength=1  InitialCondition=0  UseCircularBuffer=on
  Delay9 : Delay  InitialCondition=0  UseCircularBuffer=on
  HDL Counter6 : hdlsllib/Sources/HDL Counter  CountType=Count limited  CountInit=0  CountStep=1  CountMax=255  CountFromType=Initial value  CountFrom=0  CountResetPort=on  CountLoadPort=off  CountEnbPort=on  CountDirPort=off  CountDataType=Unsigned  CountWordLen=8  CountFracLen=0  CountSampTime=1
      settings: SourceProductBaseCode=HD
  Logical Operator1 : Logic  AllPortsSameDT=off  OutDataTypeStr=boolean
  Logical Operator4 : Logic  Operator=OR  AllPortsSameDT=off  OutDataTypeStr=boolean
  Logical Operator5 : Logic  Operator=NOT  AllPortsSameDT=off  OutDataTypeStr=boolean
  Math Function : Math  Operator=mod  RndMeth=Zero  SaturateOnIntegerOverflow=on
  Math Function1 : Math  Operator=mod  RndMeth=Zero  SaturateOnIntegerOverflow=on
  Simple Dual Port RAM : hdlsllib/HDL RAMs/Simple Dual Port RAM  ram_size=8
      settings: SourceProductName=HDL Coder  SourceProductBaseCode=HD
  Simple Dual Port RAM1 : hdlsllib/HDL RAMs/Simple Dual Port RAM  ram_size=8
      settings: SourceProductName=HDL Coder  SourceProductBaseCode=HD
  Switch1 : Switch  Criteria=u2 ~= 0
  Switch12 : Switch  Criteria=u2 > Threshold
  Switch2 : Switch  Criteria=u2 > Threshold
  Unit Delay Enabled Synchronous1 : hdlsllib/Discrete/Unit Delay Enabled Synchronous  InitialCondition=0.0  SampleTime=-1
      settings: SourceProductName=HDL Coder  SourceProductBaseCode=HD
  Unit Delay Enabled Synchronous5 : hdlsllib/Discrete/Unit Delay Enabled Synchronous  InitialCondition=0.0  SampleTime=-1
      settings: SourceProductName=HDL Coder  SourceProductBaseCode=HD
  Устранение 2pi неопределенности и вычисление разности фаз1 : Subsystem
  "Passe diff " : Outport
  wires:
  Pilot Phase/1 -> Simple Dual Port RAM/1, Simple Dual Port RAM1/1
  Logical Operator4/1 -> Simple Dual Port RAM/3, Simple Dual Port RAM1/3, HDL Counter6/2, Logical Operator5/1
  Logical Operator5/1 -> HDL Counter6/1
  "Index Pil "/1 -> Unit Delay Enabled Synchronous1/2, Logical Operator4/2
  Simple Dual Port RAM1/1 -> Устранение 2pi неопределенности и вычисление разности фаз1/1("Фаза \"левого\" пилота")
  Index Inf/1 -> Logical Operator4/1
  Simple Dual Port RAM/1 -> Устранение 2pi неопределенности и вычисление разности фаз1/2("Фаза \"правого\" пилота")
  Compare To Constant1/1 -> Logical Operator1/1
  Compare To Constant2/1 -> Logical Operator1/2
  Logical Operator1/1 -> Switch1/2
  Switch1/1 -> "Passe diff "/1
  Устранение 2pi неопределенности и вычисление разности фаз1/1("Разность фаз ") -> Switch1/1
  Constant1/1 -> Switch1/3
  Constant2/1 -> Add9/2
  ? -> Switch12/1
  ? -> Math Function/1, Unit Delay Enabled Synchronous5/1
  Delay10/1 -> ?
  Math Function/1 -> Compare To Constant8/1
  Switch12/1 -> Delay10/1
  Compare To Constant8/1 -> Switch12/2
  ? -> Unit Delay Enabled Synchronous5/2
  Add9/1 -> ?
  Unit Delay Enabled Synchronous5/1 -> Add9/1, Switch12/3
  Constant13/1 -> Math Function/2
  ? -> ?
  Delay9/1 -> Compare To Constant2/1, Compare To Constant1/1
  Constant3/1 -> Math Function1/2
  HDL Counter6/1 -> Switch2/1, Unit Delay Enabled Synchronous1/1, Math Function1/1, Simple Dual Port RAM/2, Delay9/1, Simple Dual Port RAM1/2
  Math Function1/1 -> Compare To Constant3/1
  Unit Delay Enabled Synchronous1/1 -> Switch2/3
  Compare To Constant3/1 -> Switch2/2
  Switch2/1 -> Delay1/1
  Constant4/1 -> Add1/1
  Add1/1 -> Simple Dual Port RAM1/4
  Delay1/1 -> Simple Dual Port RAM/4, Add1/2

== system OFDMTxRx2211/LTE_Detector_HDL/Подкрутка фазы1 ==
  PuuuSii : Inport
  "DifPhase " : Inport  Port=2
  Constant13 : Constant  Value=complex(0+i)  SampleTime=simParams.Ts
  Pow1 : Math  RndMeth=Zero  SaturateOnIntegerOverflow=on
  Product3 : Product
  Product4 : Product
  Unary Minus1 : UnaryMinus
  Out1 : Outport
  wires:
  PuuuSii/1 -> Product4/1
  "DifPhase "/1 -> Unary Minus1/1
  Product4/1 -> Out1/1
  Product3/1 -> Pow1/1
  Constant13/1 -> Product3/2
  Pow1/1 -> Product4/2
  Unary Minus1/1 -> Product3/1

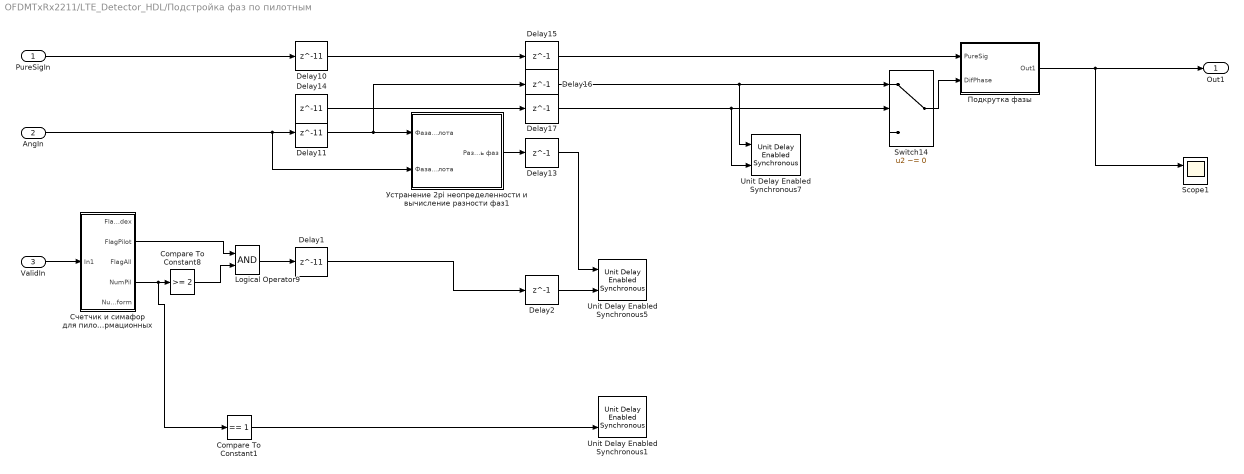
== system OFDMTxRx2211/LTE_Detector_HDL/Подстройка фаз по пилотным ==
  PureSigIn : Inport
  AngIn : Inport  Port=2
  "ValidIn " : Inport  Port=3
  Compare To Constant1 : simulink/Logic and Bit Operations/Compare To Constant  relop===  const=1  OutDataTypeStr=boolean
  Compare To Constant8 : simulink/Logic and Bit Operations/Compare To Constant  relop=>=  const=2  OutDataTypeStr=boolean
  Delay{1,10..11,14} (4 alike) : Delay  DelayLength=11  InitialCondition=0  UseCircularBuffer=on
  Delay{2,13,15..17} (5 alike) : Delay  DelayLength=1  InitialCondition=0  UseCircularBuffer=on
  Logical Operator9 : Logic  AllPortsSameDT=off  OutDataTypeStr=boolean
  Scope1 : Scope  NumInputPorts=2
  Switch14 : Switch  Criteria=u2 ~= 0
  Unit Delay Enabled Synchronous1 : hdlsllib/Discrete/Unit Delay Enabled Synchronous  InitialCondition=0.0  SampleTime=-1
      settings: SourceProductName=HDL Coder  SourceProductBaseCode=HD
  Unit Delay Enabled Synchronous5 : hdlsllib/Discrete/Unit Delay Enabled Synchronous  InitialCondition=0.0  SampleTime=-1
      settings: SourceProductName=HDL Coder  SourceProductBaseCode=HD
  Unit Delay Enabled Synchronous7 : hdlsllib/Discrete/Unit Delay Enabled Synchronous  InitialCondition=0.0  SampleTime=-1
      settings: SourceProductName=HDL Coder  SourceProductBaseCode=HD
  Подкрутка фазы : Subsystem
  Счетчик и симафор для пилотов и информационных : Subsystem
  Устранение 2pi неопределенности и вычисление разности фаз1 : Subsystem
  Out1 : Outport
  wires:
  "ValidIn "/1 -> Счетчик и симафор для пилотов и информационных/1(In1)
  Delay10/1 -> Delay15/1
  Подкрутка фазы/1(Out1) -> Scope1/1, Out1/1
  PureSigIn/1 -> Delay10/1
  Delay11/1 -> Устранение 2pi неопределенности и вычисление разности фаз1/1("Фаза \"левого\" пилота"), Delay16/1
  Switch14/1 -> Подкрутка фазы/2("DifPhase ")
  Устранение 2pi неопределенности и вычисление разности фаз1/1("Разность фаз ") -> Delay13/1
  Delay16/1 -> Unit Delay Enabled Synchronous7/1, Switch14/1
  Delay15/1 -> Подкрутка фазы/1(PureSig)
  AngIn/1 -> Устранение 2pi неопределенности и вычисление разности фаз1/2("Фаза \"правого\" пилота"), Delay11/1
  Delay13/1 -> Unit Delay Enabled Synchronous5/1
  Delay17/1 -> Unit Delay Enabled Synchronous7/2, Switch14/2
  Delay14/1 -> Delay17/1
  Счетчик и симафор для пилотов и информационных/4(NumPil) -> Compare To Constant1/1, Compare To Constant8/1
  Compare To Constant8/1 -> Logical Operator9/2
  Счетчик и симафор для пилотов и информационных/2(FlagPilot) -> Logical Operator9/1
  Logical Operator9/1 -> Delay1/1
  Delay1/1 -> Delay2/1
  Delay2/1 -> Unit Delay Enabled Synchronous5/2
  Compare To Constant1/1 -> Unit Delay Enabled Synchronous1/2

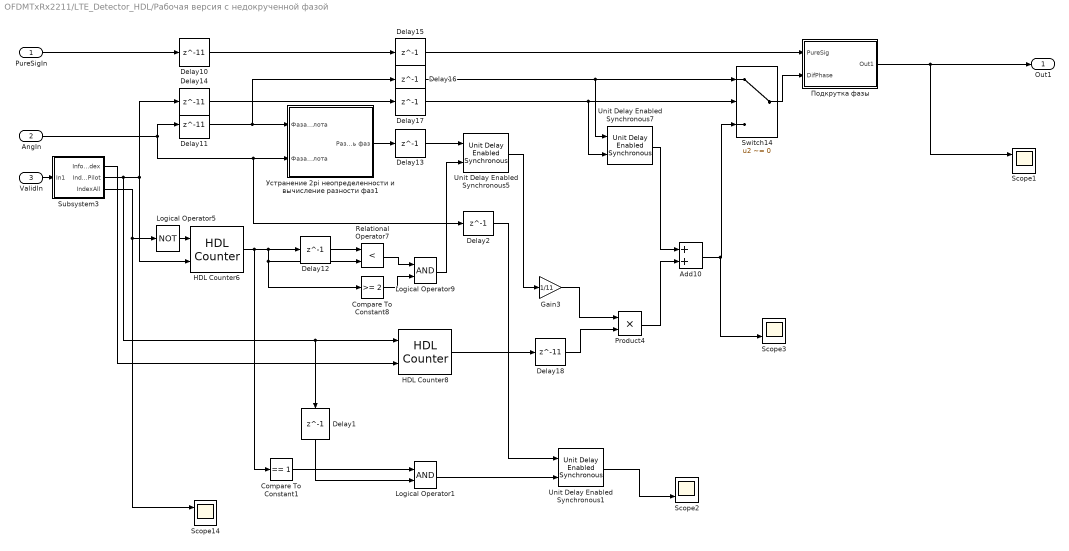
== system OFDMTxRx2211/LTE_Detector_HDL/Рабочая версия с недокрученной фазой  ==
  PureSigIn : Inport
  AngIn : Inport  Port=2
  "ValidIn " : Inport  Port=3
  Add10 : Sum  Inputs=2
  Compare To Constant1 : simulink/Logic and Bit Operations/Compare To Constant  relop===  const=1  OutDataTypeStr=boolean
  Compare To Constant8 : simulink/Logic and Bit Operations/Compare To Constant  relop=>=  const=2  OutDataTypeStr=boolean
  Delay{1..2,12..13,15..17} (7 alike) : Delay  DelayLength=1  InitialCondition=0  UseCircularBuffer=on
  Delay{10..11,14,18} (4 alike) : Delay  DelayLength=11  InitialCondition=0  UseCircularBuffer=on
  Gain3 : Gain  Gain=1/11
  HDL Counter6 : hdlsllib/Sources/HDL Counter  CountType=Count limited  CountInit=0  CountStep=1  CountMax=20  CountFromType=Initial value  CountFrom=0  CountResetPort=on  CountLoadPort=off  CountEnbPort=on  CountDirPort=off  CountDataType=Unsigned  CountWordLen=8  CountFracLen=0  CountSampTime=1
      settings: SourceProductBaseCode=HD
  HDL Counter8 : hdlsllib/Sources/HDL Counter  CountType=Count limited  CountInit=1  CountStep=1  CountMax=20  CountFromType=Initial value  CountFrom=1  CountResetPort=on  CountLoadPort=off  CountEnbPort=on  CountDirPort=off  CountDataType=Unsigned  CountWordLen=8  CountFracLen=0  CountSampTime=1
      settings: SourceProductBaseCode=HD
  Logical Operator1 : Logic  AllPortsSameDT=off  OutDataTypeStr=boolean
  Logical Operator5 : Logic  Operator=NOT  AllPortsSameDT=off  OutDataTypeStr=boolean
  Logical Operator9 : Logic  AllPortsSameDT=off  OutDataTypeStr=boolean
  Product4 : Product
  Relational Operator7 : RelationalOperator  Operator=<  OutDataTypeStr=boolean  RndMeth=Nearest
  Scope{1..3,14} (4 alike) : Scope  NumInputPorts=2
  Subsystem3 : Subsystem
  Switch14 : Switch  Criteria=u2 ~= 0
  Unit Delay Enabled Synchronous1 : hdlsllib/Discrete/Unit Delay Enabled Synchronous  InitialCondition=0.0  SampleTime=-1
      settings: SourceProductName=HDL Coder  SourceProductBaseCode=HD
  Unit Delay Enabled Synchronous5 : hdlsllib/Discrete/Unit Delay Enabled Synchronous  InitialCondition=0.0  SampleTime=-1
      settings: SourceProductName=HDL Coder  SourceProductBaseCode=HD
  Unit Delay Enabled Synchronous7 : hdlsllib/Discrete/Unit Delay Enabled Synchronous  InitialCondition=0.0  SampleTime=-1
      settings: SourceProductName=HDL Coder  SourceProductBaseCode=HD
  Подкрутка фазы : Subsystem
  Устранение 2pi неопределенности и вычисление разности фаз1 : Subsystem
  Out1 : Outport
  wires:
  "ValidIn "/1 -> Subsystem3/1(In1)
  Delay10/1 -> Delay15/1
  Подкрутка фазы/1(Out1) -> Scope1/1, Out1/1
  PureSigIn/1 -> Delay10/1
  Delay11/1 -> Устранение 2pi неопределенности и вычисление разности фаз1/1("Фаза \"левого\" пилота"), Delay16/1
  Switch14/1 -> Подкрутка фазы/2("DifPhase ")
  Subsystem3/2(IndexPilot) -> HDL Counter8/1, Delay1/1, Delay14/1, HDL Counter6/2
  Logical Operator9/1 -> Unit Delay Enabled Synchronous5/2
  Устранение 2pi неопределенности и вычисление разности фаз1/1("Разность фаз ") -> Delay13/1
  Relational Operator7/1 -> Logical Operator9/1
  Delay16/1 -> Unit Delay Enabled Synchronous7/1, Switch14/1
  Subsystem3/3(IndexAll) -> Scope14/1, Logical Operator5/1
  Delay15/1 -> Подкрутка фазы/1(PureSig)
  Delay12/1 -> Relational Operator7/1
  AngIn/1 -> Delay2/1, Устранение 2pi неопределенности и вычисление разности фаз1/2("Фаза \"правого\" пилота"), Delay11/1
  Logical Operator5/1 -> HDL Counter6/1
  HDL Counter8/1 -> Delay18/1
  Delay13/1 -> Unit Delay Enabled Synchronous5/1
  Compare To Constant8/1 -> Logical Operator9/2
  Unit Delay Enabled Synchronous5/1 -> Gain3/1
  Subsystem3/1(InformIndex) -> HDL Counter8/2
  Product4/1 -> Add10/2
  Gain3/1 -> Product4/1
  Delay17/1 -> Unit Delay Enabled Synchronous7/2, Switch14/2
  Delay18/1 -> Product4/2
  Delay14/1 -> Delay17/1
  Add10/1 -> Scope3/2, Switch14/3
  Unit Delay Enabled Synchronous7/1 -> Add10/1
  Delay2/1 -> Unit Delay Enabled Synchronous1/1
  Logical Operator1/1 -> Unit Delay Enabled Synchronous1/2
  Compare To Constant1/1 -> Logical Operator1/1
  HDL Counter6/1 -> Compare To Constant1/1, Delay12/1, Relational Operator7/2, Compare To Constant8/1
  Delay1/1 -> Logical Operator1/2
  Unit Delay Enabled Synchronous1/1 -> Scope2/2

== system OFDMTxRx2211/LTE_Detector_HDL/Стробирование сигнала на nFFT отсчетов ==
  In1 : Inport
  In2 : Inport  Port=2
  Compare To Constant : simulink/Logic and Bit Operations/Compare To Constant  relop=>  const=0  OutDataTypeStr=boolean
  Delay1 : Delay  DelayLength=1  InitialCondition=0
  Delay2 : Delay  DelayLength=2428  InitialCondition=0
  HDL Counter : hdlsllib/Sources/HDL Counter  CountType=Count limited  CountInit=0  CountStep=1  CountMax=1023  CountFromType=Initial value  CountFrom=0  CountResetPort=off  CountLoadPort=off  CountEnbPort=on  CountDirPort=off  CountDataType=Unsigned  CountWordLen=11  CountFracLen=0  CountSampTime=1
      settings: SourceProductBaseCode=HD
  Logical Operator1 : Logic  IconShape=distinctive  AllPortsSameDT=off  OutDataTypeStr=boolean
  Logical Operator4 : Logic  Operator=OR  IconShape=distinctive  AllPortsSameDT=off  OutDataTypeStr=boolean
  dataOut : Outport
  ValidOut : Outport  Port=2
  wires:
  Logical Operator4/1 -> Delay1/1, HDL Counter/1, ValidOut/1
  In1/1 -> Delay2/1
  HDL Counter/1 -> Compare To Constant/1
  Logical Operator1/1 -> Logical Operator4/2
  Delay1/1 -> Logical Operator1/2
  Compare To Constant/1 -> Logical Operator1/1
  Delay2/1 -> dataOut/1
  In2/1 -> Logical Operator4/1

== system OFDMTxRx2211/LTE_Detector_HDL/Устранение 2pi неопределенности и вычисление разности фаз ==
  "Фаза \"левого\" пилота" : Inport
  "Фаза \"правого\" пилота" : Inport  Port=2
  Add8 : Sum  Inputs=+-
  Add9 : Sum  Inputs=-+
  Constant8 : Constant  Value=3.1416*2  OutDataTypeStr=double  SampleTime=simParams.Ts
  Relational Operator7 : RelationalOperator  Operator=>  OutDataTypeStr=boolean  RndMeth=Nearest
  Switch10 : Switch  Criteria=u2 ~= 0
  "Разность фаз " : Outport
  wires:
  Switch10/1 -> Add9/2
  Add8/1 -> Switch10/1
  "Фаза \"правого\" пилота"/1 -> Switch10/3, Relational Operator7/1, Add8/1
  Constant8/1 -> Add8/2
  "Фаза \"левого\" пилота"/1 -> Add9/1, Relational Operator7/2
  Relational Operator7/1 -> Switch10/2
  Add9/1 -> "Разность фаз "/1

== system OFDMTxRx2211/LTE_Detector_HDL/Устранение 2pi неопределенности и вычисление разности фаз2 ==
  "Фаза \"левого\" пилота" : Inport
  "Фаза \"правого\" пилота" : Inport  Port=2
  Enable : EnablePort
  Add8 : Sum  Inputs=+-
  Add9 : Sum  Inputs=-+
  Constant8 : Constant  Value=3.1416*2  OutDataTypeStr=double  SampleTime=simParams.Ts
  Relational Operator7 : RelationalOperator  Operator=>  OutDataTypeStr=boolean  RndMeth=Nearest
  Switch10 : Switch  Criteria=u2 ~= 0
  "Разность фаз " : Outport
  wires:
  Switch10/1 -> Add9/2
  Add8/1 -> Switch10/1
  "Фаза \"правого\" пилота"/1 -> Switch10/3, Relational Operator7/1, Add8/1
  Constant8/1 -> Add8/2
  "Фаза \"левого\" пилота"/1 -> Add9/1, Relational Operator7/2
  Relational Operator7/1 -> Switch10/2
  Add9/1 -> "Разность фаз "/1

== system OFDMTxRx2211/DUT/symmetric /Add CP and windowing ==
  In1 : Inport
  In2 : Inport  Port=2
  Compare To Constant : simulink/Logic and Bit Operations/Compare To Constant  relop=>=  const=896  OutDataTypeStr=boolean
  Delay1 : Delay  DelayLength=1024
  Delay2 : Delay  DelayLength=1024
  FFT : Subsystem
  HDL Counter : hdlsllib/Sources/HDL Counter  CountType=Count limited  CountInit=0  CountStep=1  CountMax=1023  CountFromType=Initial value  CountFrom=0  CountResetPort=on  CountLoadPort=off  CountEnbPort=on  CountDirPort=off  CountDataType=Unsigned  CountWordLen=10  CountFracLen=0  CountSampTime=1
      settings: SourceProductBaseCode=HD
  Logical Operator2 : Logic  Operator=NOT  AllPortsSameDT=off  OutDataTypeStr=boolean
  Scope : Scope
  Switch1 : Switch  Criteria=u2 > Threshold
  y_out2 : Scope  NumInputPorts=3
  Out1 : Outport
  wires:
  Delay1/1 -> y_out2/2, Switch1/3
  HDL Counter/1 -> Compare To Constant/1
  Compare To Constant/1 -> Switch1/2
  Logical Operator2/1 -> HDL Counter/1
  Switch1/1 -> FFT/1(dataIn), y_out2/1, Out1/1
  In1/1 -> Delay1/1, Switch1/1
  In2/1 -> Delay2/1, Logical Operator2/1, HDL Counter/2
  Delay2/1 -> FFT/2(validIn), y_out2/3
  FFT/1(dataOut) -> Scope/1

== system OFDMTxRx2211/DUT/symmetric /IFFT ==
  note: Set input of FFT to input wordlength + FFT growth to allow
      | the output of the FFT to scale. Maximum bit growth is equal
      | to log2(nFFT).
  dataIn : Inport
  validIn : Inport  Port=2
  Data Type Conversion : DataTypeConversion  OutDataTypeStr=fixdt(1,23,15)  RndMeth=Nearest
  Delay{1..2,4..5} (4 alike) : Delay  DelayLength=1  InitialCondition=0  InputProcessing=Columns as channels (frame based)
  IFFT HDL Optimized : dspxfrm3/IFFT HDL Optimized  FFTLength=simParams.nFFT  Architecture=Streaming Radix 2^2  ComplexMultiplication=Use 3 multipliers and 5 adders  BitReversedOutput=off  BitReversedInput=off  Normalize=on  SimulateUsing=Code generation  RoundingMethod=Floor  ResetInputPort=off  StartOutputPort=off  EndOutputPort=off
      settings: SourceProductName=DSP System Toolbox  SourceProductBaseCode=DS
  Signal Specification : SignalSpecification  Dimensions=1
  Signal Specification1 : SignalSpecification  Dimensions=1
  dataOut : Outport
  validOut : Outport  Port=2
  wires:
  validIn/1 -> Delay2/1
  dataIn/1 -> Delay1/1
  Delay4/1 -> dataOut/1
  Delay2/1 -> Signal Specification1/1
  IFFT HDL Optimized/1 -> Delay4/1
  IFFT HDL Optimized/2 -> Delay5/1
  Signal Specification/1 -> IFFT HDL Optimized/1
  Signal Specification1/1 -> IFFT HDL Optimized/2
  Data Type Conversion/1 -> Signal Specification/1
  Delay1/1 -> Data Type Conversion/1
  Delay5/1 -> validOut/1
